simulink model "Project_microgrid_2016"  (R2016a)
settings: Solver=VariableStepAuto  SolverMode=SingleTasking  StartTime=0.0  StopTime=0.3  RelTol=1e-3
undefined symbols (not defined in the file): D1, D11, Delta, DiscIntNeverNeededParam, find_system, Hydride, Metal, Nickel
libraries: powerlib x77, powerlib_meascontrol x31, sps_avr x7, simulink_extras x4, simulink x3, electricdrivelib x1, spsDieselMotorModel x1, re_lib x1
(part 3 of 5)

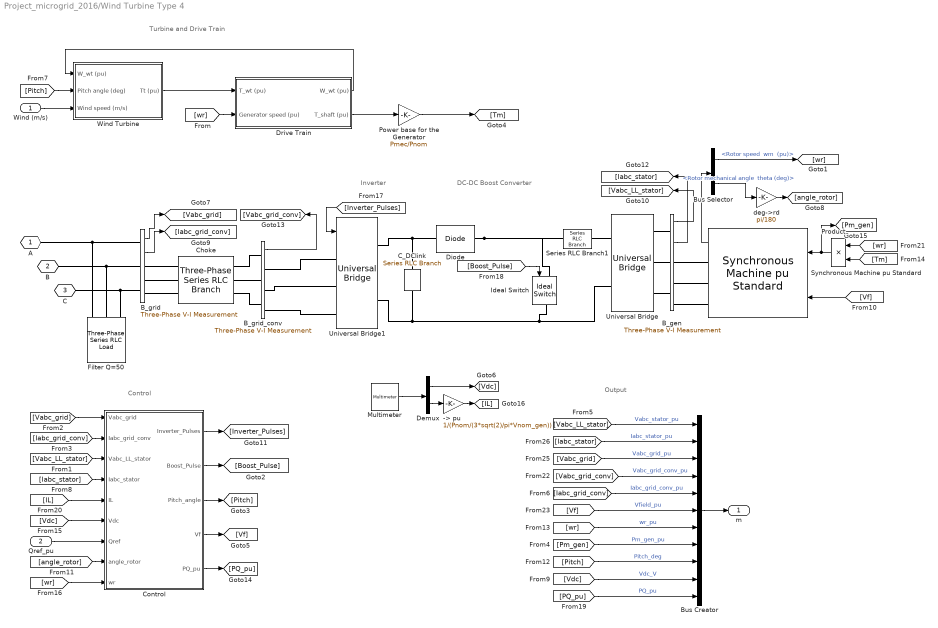
== system Project_microgrid_2016/Wind Turbine Type 4 ==
  note: Turbine and Drive Train
  note: Control
  note: Inverter
  note: DC-DC Boost Converter
  note: Output
  "Wind (m/s) " : Inport
  Qref_pu : Inport  Port=2
  -> pu : Gain  Gain=1/(Pnom/(3*sqrt(2)/pi*Vnom_gen))  SaturateOnIntegerOverflow=on  OutDataTypeStr=Inherit: Same as input  ParamDataTypeStr=Inherit: Same as input
  B_gen : powerlib/Measurements/Three-Phase V-I Measurement  VoltageMeasurement=phase-to-phase  SetLabelV=off  LabelV=Vabc  Vpu=on  VpuLL=off  CurrentMeasurement=yes  SetLabelI=off  LabelI=Iabc  Ipu=on  Pbase=Pnom  Vbase=Vnom_gen  OutputType=Complex  PhasorSimulation=off  PSBequivalent=0
  B_grid : powerlib/Measurements/Three-Phase V-I Measurement  VoltageMeasurement=phase-to-ground  SetLabelV=off  LabelV=Vabc  Vpu=on  VpuLL=off  CurrentMeasurement=yes  SetLabelI=off  LabelI=Iabc  Ipu=on  Pbase=Pnom  Vbase=Vnom  OutputType=Complex  PhasorSimulation=off  PSBequivalent=0
  B_grid_conv : powerlib/Measurements/Three-Phase V-I Measurement  VoltageMeasurement=phase-to-ground  SetLabelV=off  LabelV=Vabc  Vpu=on  VpuLL=off  CurrentMeasurement=no  SetLabelI=off  LabelI=Iabc  Ipu=on  Pbase=Pnom  Vbase=Vnom  OutputType=Complex  PhasorSimulation=off  PSBequivalent=0
  Bus Creator : BusCreator  Inputs=11
  Bus Selector : BusSelector  OutputSignals="Mechanical.Rotor speed  wm  (pu),Mechanical.Rotor mechanical angle  theta (deg)"
  C_DClink : powerlib/Elements/Series RLC Branch  LConnTagsString=__new0  RConnTagsString=__new0  BranchType=C  Resistance=1  Inductance=1e-3  SetiL0=off  InitialCurrent=0  Capacitance=C_DClink  Setx0=on  InitialVoltage=Vdc_nom  Measurements=Branch voltage
  "Choke " : powerlib/Elements/Three-Phase Series RLC Branch  LConnTagsString=A|B|C  RConnTagsString=A|B|C  BranchType=RL  Resistance=R_RL*Vnom^2/Pnom  Inductance=L_RL*Vnom^2/Pnom/(2*pi*Fnom)  Capacitance=[]  Measurements=None
  Control : Subsystem
  Demux : Demux  Outputs=2
  Diode : powerlib/Power Electronics/Diode  Ron=1e-6/Nb_wt  Lon=0  Vf=0  IC=0  UseSnubber=off  Rs=inf  Cs=inf  Measurements=off
  Drive Train : Subsystem  mask(Wind Turbine shaft){H_WT=H_WT, Ksh=Ksh, D_mutual=D_mutual, wbase=2*pi*Fnom/p, w_wt0=w_wt0, torque0=torque0, Ts=Ts}
      mask prompts: H_WT "Wind turbine inertia constant H (s):"; Ksh "Shaft spring constant (pu of nominal mechanical torque/rad):"; D_mutual "Shaft mutual damping (pu of nominal mechanical torque/pu dw):"; wbase "Shaft base speed (rad/s):"; w_wt0 "Turbine initial speed (pu of base speed):"; torque0 "Initial output torque (pu of nominal mechanical torque):"; Ts "Sample time (s):"
      mask help:
      | This block implements a wind turbine drive train model. All shaft parameters are referred to high-speed shaft (generator shaft).
      |
      | The first input is the wind turbine torque in per unit (pu) based on the nominal power of the turbine and the base speed of the generator. The second input is the generator speed in pu based on the base speed of the generator.
      |
      | The outputs are:
      | 1- the transmitted torque of the shaft in pu based on the nominal power of the turbine and the base speed of the generator.
      | 2- the wind turbine speed in pu of the base speed of the generator.
  Filter Q=50 : powerlib/Elements/Three-Phase Series RLC Load  LConnTagsString=A|B|C  Configuration=Y (grounded)  NominalVoltage=Vnom  Vabc=[1e3 1e3 1e3]  Vabcp=[1e3 1e3 1e3]  NominalFrequency=Fnom  UnbalancedPower=off  ActivePower=C_var_filter/Q_filter  InductivePower=0  CapacitivePower=C_var_filter  Pabc=[10e3 9e3 11e3]  QLabc=[100 90 110]  QCabc=[100 90 110]  Pabcp=[10e3 9e3 11e3]  QLabcp=[100 90 110]  QCabcp=[100 90 110]  Measurements=None  LoadType=constant Z
  Ideal Switch : powerlib/Power Electronics/Ideal Switch  Ron=1e-6/Nb_wt  Lon=0  IC=0  Rs=1e5/Nb_wt  Cs=inf  Measurements=off
  Multimeter : powerlib/Measurements/Multimeter  PhasorSimulation=off  OutputType=Complex  sel=[2 3]  L=3  Gain=[1 1]  yselected={'Ub: Wind Turbine Type 4/C_DClink','Ib: Wind Turbine Type 4/Series RLC Branch1'};  PSBOutputType=1  PSBequivalent=0  AxesSetting=[0,0.1,-100,100]  Display=0  SavedBlockNames=-11
  Power base for the Generator : Gain  Gain=Pmec/Pnom  SaturateOnIntegerOverflow=on  OutDataTypeStr=Inherit: Same as input  ParamDataTypeStr=Inherit: Same as input
  Product : Product  RndMeth=Zero
  Series RLC Branch1 : powerlib/Elements/Series RLC Branch  LConnTagsString=__new0  RConnTagsString=__new0  BranchType=RL  Resistance=R_Boost  Inductance=L_Boost  SetiL0=off  InitialCurrent=0  Capacitance=1.0  Setx0=off  InitialVoltage=0  Measurements=Branch current
  Synchronous Machine pu Standard : powerlib/Machines/Synchronous Machine pu Standard  PresetModel=No  MechanicalLoad=Mechanical power Pm  ShowDetailedParameters=on  RotorType=Salient-pole  Units=per unit standard parameters  MeasurementBus=off  NominalParameters="[ Pnom  Vnom_gen Fnom ]"  Reactances1=[ 1.81, 0.3, 0.23, 1.76, 0.65, 0.25, 0.15 ]  Reactances2="[ Xd, Xd1, Xd2, Xq,  Xq2,  Xl ]"  dAxisTimeConstants=Open-circuit  qAxisTimeConstants=Short-circuit  TimeConstants1="[ 4.4849  0.0681  0.1  ]"  TimeConstants2=[ 8.0, 0.03, 1.0, 0.07 ]  TimeConstants3="[  Tdo1  Tdo2  Tq2  ]"  TimeConstants4=[ 8.0, 0.03, 0.3371, 0.0295 ]  TimeConstants5=[ 1.01, 0.053, 0.1 ]  TimeConstants6=[ 1.3201, 0.023, 1.0, 0.07 ]  TimeConstants7="[  1.01  0.053  0.051266  ]"  TimeConstants8=[ 1.3201, 0.0231, 0.3371, 0.0295 ]  StatorResistance=Resistance  Mechanical=[ H F p]  PolePairs=1  InitialConditions=init  SetSaturation=off  Saturation=[0.6404,0.7127,0.8441,0.9214,0.9956,1.082,1.19,1.316,1.457;0.7,0.7698,0.8872,0.9466,0.9969,1.046,1.1,1.151,1.201]  LoadFlowParameters=[1,0,0,0,0]  TsPowergui=0  TsBlock=-1  IterativeModel=Trapezoidal non iterative  IterativeDiscreteModel=Trapezoidal non iterative  BusType=PV  Pref=0  Qref=0  Qmin=-inf  Qmax=inf  PLF=0  QLF=0
  Universal Bridge : powerlib/Power Electronics/Universal Bridge  Arms=3  SnubberResistance=2*Ts_snub/(Pnom/(1000*2*pi*Fnom*Vnom_gen^2))  SnubberCapacitance=Pnom/(1000*2*pi*Fnom*Vnom_gen^2)  Device=Diodes  Ron=1e-6/Nb_wt  Lon=0  ForwardVoltages="[  0  0  ]"  ForwardVoltage=0  GTOparameters=[ 10e-6 , 20e-6 ]  IGBTparameters=[ 1e-6 , 2e-6 ]  Measurements=None  Measurements_2=None  converterType=Rectifier
  Universal Bridge1 : powerlib/Power Electronics/Universal Bridge  Arms=3  SnubberResistance=1e6/Nb_wt  SnubberCapacitance=inf  Device=IGBT / Diodes  Ron=1e-6/Nb_wt  Lon=0  ForwardVoltages="[  0  0  ]"  ForwardVoltage=0  GTOparameters=[ 10e-6 , 20e-6 ]  IGBTparameters=[ 1e-6 , 2e-6 ]*0  Measurements=None  Measurements_2=None  converterType=Rectifier
  Wind Turbine : Subsystem  mask(Wind Turbine){Prated=Pmec, c1_c8=c1_c8, K1_K2=K1_K2, wind0=wind0, Ts=Ts}
      mask prompts: Prated "Nominal mechanical output power (W):"; c1_c8 "Coefficients [c1 ... c8]"; K1_K2 "Parameters [K1 K2]"; wind0 "Initial wind speed (m/s):"; Ts "Sample time (s):"
      mask help:
      | This block implements a generic wind turbine models.
      |
      | The first input is the turbine speed in per unit of the generator base speed. For a synchronous or asynchronous generator, the base speed is the synchronous speed. For a permanent-magnet generator, the base speed is defined as the speed producing nominal voltage at  no load. The second input is the blade pitch angle in degrees. The third input is the wind speed in m/s.
      |
      | The output is the torque applied to the drive train in per unit based on the nominal power of the turbine and the base speed of the generator.
      mask init:
      | c1 = c1_c8(1);
      | c2 = c1_c8(2);
      | c3 = c1_c8(3);
      | c4 = c1_c8(4);
      | c5 = c1_c8(5);
      | c6 = c1_c8(6);
      | c7 = c1_c8(7);;
      | c8 = c1_c8(8);
      | 
      | K1=K1_K2(1);
      | K2=K1_K2(2);
      settings: OpenFcn=power_openblockproxy();
      mask Display: disp('');
  deg->rd : Gain  Gain=pi/180  SaturateOnIntegerOverflow=on  OutDataTypeStr=Inherit: Same as input  ParamDataTypeStr=Inherit: Same as input
  A : PMIOPort  Tag=PMCPort  Side=Left
  B : PMIOPort  Tag=PMCPort  Port=2  Side=Left
  C : PMIOPort  Tag=PMCPort  Port=3  Side=Left
  m : Outport
  wires:
  [Vf] -> Synchronous Machine pu Standard/2
  Wind Turbine/1(Tt (pu)) -> Drive Train/1(T_wt (pu))
  [wr] -> Drive Train/2(Generator speed (pu))
  Drive Train/2(T_shaft (pu)) -> Power base for the Generator/1
  Power base for the Generator/1 -> [Tm]
  "Wind (m/s) "/1 -> Wind Turbine/3(Wind speed (m/s))
  Drive Train/1(W_wt (pu)) -> Wind Turbine/1(W_wt (pu))
  [Pitch] -> Wind Turbine/2(Pitch angle (deg))
  Bus Selector/2 -> deg->rd/1  "<Rotor mechanical angle  theta (deg)>"
  deg->rd/1 -> [angle_rotor]
  Bus Selector/1 -> [wr]  "<Rotor speed  wm  (pu)>"
  [wr] -> Product/1
  Synchronous Machine pu Standard/1 -> Bus Selector/1
  B_grid_conv/1 -> [Vabc_grid_conv]
  [Tm] -> Product/2
  Product/1 -> Synchronous Machine pu Standard/1, [Pm_gen]
  B_grid/1 -> [Vabc_grid]
  B_grid/2 -> [Iabc_grid_conv]
  B_gen/1 -> [Vabc_LL_stator]
  B_gen/2 -> [Iabc_stator]
  [Vabc_grid] -> Control/1(Vabc_grid)
  [Iabc_grid_conv] -> Control/2(Iabc_grid_conv)
  [Vabc_LL_stator] -> Control/3(Vabc_LL_stator)
  [Iabc_stator] -> Control/4(Iabc_stator)
  [Vdc] -> Control/6(Vdc)
  Qref_pu/1 -> Control/7(Qref)
  [angle_rotor] -> Control/8(angle_rotor)
  [wr] -> Control/9(wr)
  Control/1(Inverter_Pulses) -> [Inverter_Pulses]
  Control/2(Boost_Pulse) -> [Boost_Pulse]
  Control/3(Pitch_angle) -> [Pitch]
  Control/4(Vf) -> [Vf]
  [Inverter_Pulses] -> Universal Bridge1/1
  [Boost_Pulse] -> Ideal Switch/1
  Control/5(PQ_pu) -> [PQ_pu]
  [Vabc_LL_stator] -> Bus Creator/1  "Vabc_stator_pu"
  [Iabc_stator] -> Bus Creator/2  "Iabc_stator_pu"
  [Vabc_grid] -> Bus Creator/3  "Vabc_grid_pu"
  Bus Creator/1 -> m/1
  [Vabc_grid_conv] -> Bus Creator/4  "Vabc_grid_conv_pu"
  [Iabc_grid_conv] -> Bus Creator/5  "Iabc_grid_conv_pu"
  [Vf] -> Bus Creator/6  "Vfield_pu"
  [wr] -> Bus Creator/7  "wr_pu"
  [Pm_gen] -> Bus Creator/8  "Pm_gen_pu"
  [Pitch] -> Bus Creator/9  "Pitch_deg"
  [Vdc] -> Bus Creator/10  "Vdc_V"
  [PQ_pu] -> Bus Creator/11  "PQ_pu"
  [IL] -> Control/5(IL)
  Multimeter/1 -> Demux/1
  Demux/1 -> [Vdc]
  Demux/2 -> -> pu/1
  -> pu/1 -> [IL]
  connections:
  B_grid/RConn1 -- "Choke "/LConn1
  B_grid/RConn2 -- "Choke "/LConn2
  B_grid/RConn3 -- "Choke "/LConn3
  A/RConn1 -- B_grid/LConn1 -- Filter Q=50/LConn1
  Filter Q=50/LConn2 -- B_grid/LConn2 -- B/RConn1
  Filter Q=50/LConn3 -- B_grid/LConn3 -- C/RConn1
  "Choke "/RConn1 -- B_grid_conv/LConn1
  "Choke "/RConn2 -- B_grid_conv/LConn2
  "Choke "/RConn3 -- B_grid_conv/LConn3
  Series RLC Branch1/LConn1 -- Universal Bridge/RConn1
  Universal Bridge/LConn1 -- B_gen/LConn1
  Universal Bridge/LConn2 -- B_gen/LConn2
  Universal Bridge/LConn3 -- B_gen/LConn3
  Diode/LConn1 -- Series RLC Branch1/RConn1 -- Ideal Switch/LConn1
  Universal Bridge1/RConn1 -- Diode/RConn1 -- C_DClink/LConn1
  Universal Bridge/RConn2 -- Universal Bridge1/RConn2 -- C_DClink/RConn1 -- Ideal Switch/RConn1
  Synchronous Machine pu Standard/RConn3 -- B_gen/RConn3
  Synchronous Machine pu Standard/RConn2 -- B_gen/RConn2
  Synchronous Machine pu Standard/RConn1 -- B_gen/RConn1
  B_grid_conv/RConn2 -- Universal Bridge1/LConn2
  B_grid_conv/RConn1 -- Universal Bridge1/LConn1
  B_grid_conv/RConn3 -- Universal Bridge1/LConn3

== system Project_microgrid_2016/Battery/Subsystem4 ==
  "  " : powerlib/Measurements/Voltage Measurement  PhasorSimulation=off  OutputType=Complex  PSBequivalent=0
  "    " : powerlib/Elements/Series RLC Branch  LConnTagsString=__new0  RConnTagsString=__new0  BranchType=RC  Resistance=0  Inductance=69e-3  SetiL0=off  InitialCurrent=0  Capacitance=9.6e-7  Setx0=off  InitialVoltage=0  Measurements=None
  " Measurement" : powerlib/Measurements/Voltage Measurement  PhasorSimulation=off  OutputType=Complex  PSBequivalent=0
  " Measurement1" : powerlib/Measurements/Current Measurement  PhasorSimulation=off  OutputType=Complex  PSBequivalent=0
  Diode : powerlib/Power Electronics/Diode  Ron=0.001  Lon=0  Vf=0.8  IC=0  UseSnubber=off  Rs=500  Cs=250e-9  Measurements=on
  Mosfet : powerlib/Power Electronics/Mosfet  Ron=0.1  Lon=0  Rd=0.01  Vfd=0  IC=0  Rs=1e5  Cs=inf  Measurements=on
  Pulse Generator : DiscretePulseGenerator  PulseType=Time based  Period=1/100000  PulseWidth=50
  Scope : Scope  NumInputPorts=2
  Series RLC Branch : powerlib/Elements/Series RLC Branch  LConnTagsString=__new0  RConnTagsString=__new0  BranchType=RL  Resistance=0  Inductance=2.332e-3  SetiL0=off  InitialCurrent=0  Capacitance=1e-6  Setx0=off  InitialVoltage=0  Measurements=None
  + : PMIOPort  Side=Left
  _ : PMIOPort  Port=2  Side=Left
  ++ : PMIOPort  Port=3  Side=Right
  __ : PMIOPort  Port=4  Side=Right
  wires:
  Pulse Generator/1 -> Mosfet/1
  "  "/1 -> Scope/1
  " Measurement"/1 -> Scope/2
  connections:
  "  "/LConn1 -- Series RLC Branch/LConn1 -- +/RConn1
  Diode/RConn1 -- " Measurement1"/LConn1 -- "    "/LConn1
  ++/RConn1 -- " Measurement"/LConn1 -- " Measurement1"/RConn1
  Mosfet/RConn1 -- _/RConn1 -- "  "/LConn2 -- "    "/RConn1 -- __/RConn1 -- " Measurement"/LConn2
  Series RLC Branch/RConn1 -- Mosfet/LConn1 -- Diode/LConn1

== system Project_microgrid_2016/Diesle Generator/EXCITATION ==
  Vref : Inport
  Vt : Inport  Port=2
  It : Inport  Port=3
  Ifd : Inport  Port=4
  Vstab : Inport  Port=5
  AC1A : Subsystem  VariantControl=Variant1
  AC4A : Subsystem  VariantControl=Variant2
  AC5A : Subsystem  VariantControl=Variant3
  DC1A : Subsystem  VariantControl=Variant4
  DC2A : Subsystem  VariantControl=Variant5
  ST1A : Subsystem  VariantControl=Variant6
  ST2A : sps_avr/ST2A Excitation System  VariantControl=Variant7  Tr=20e-3  KaTa=[120 0.15]  VRminmax=[0 1.0]  KfTf=[0.05 1.0]  KeTe=[1.0 0.5]  KI=8.0  Kp=4.88  Xd=1.56  Kc=1.82  v0=[1,1.42734]  I0=0.2739  TsBlock=-2
  Efd : Outport

== system Project_microgrid_2016/Inveter/VSC Contoler ==
  VSC Control : Subsystem  mask(VSC Main Controller){nom=[ 7500  50 ], Vnom=[ 25e3 260 ], Vnom_dc=600, RLxfo=[0.002  0.06 ], RLchoke=[2e-3  250e-6  ], K_VDCreg=[7  800], K_Ireg=[0.3 20], Ts=0.0001}
      mask prompts: nom "Nominal power and frequency [ Pnom(VA)  Fnom(Hz) ]:"; Vnom "Nominal primary and secondary voltages (Vrms LL) [ Vnom_prim   Vnom_sec ]:"; Vnom_dc "Nominal DC bus voltage (V):"; RLxfo "Total transformer leakage impedance (pu/Pnom) [ Rxfo  Lxf ]"; RLchoke "Choke impedance [ R(ohm) L(H) ]"; K_VDCreg "VDC regultator gains [ Kp  Ki ]:"; K_Ireg "Current regulator gains [ Kp  Ki ]:"; Ts "Sample time"
      mask init:
      | Pnom=nom(1);
      | Fnom=nom(2);
      | Vnom_prim=Vnom(1);
      | Vnom_sec=Vnom(2);
      | Zbase=Vnom_sec^2/Pnom;
      | Rtot_pu=RLxfo(1) + RLchoke(1)/Zbase;
      | Ltot_pu=RLxfo(2) + RLchoke(2)/(Zbase/(2*pi*Fnom));
      | Kp_VDCreg=K_VDCreg(1);
      | Ki_VDCreg=K_VDCreg(2);
      | Kp_Ireg=K_Ireg(1);
      | Ki_Ireg=K_Ireg(2);
      | Vdc_ref=Vnom_dc;
      | % Used to determine initial value of Boost Control (MPPT)
      | assignin('base','Vdc_ref_Inv',Vdc_ref);
  Inveter Pulse : Outport
  wires:
  [Vabc_B1] -> VSC Control/1(Vabc_prim)
  [Iabc_B1] -> VSC Control/2(Iabc_prim)
  [Vdc] -> VSC Control/3(Vdc_mes)
  VSC Control/1(Pulses) -> Inveter Pulse/1

== system Project_microgrid_2016/Relay G/AC Time Overcurrent Relay2 ==
  I : Inport
  Clock : Clock
  Irms : powerlib_meascontrol/Measurements/RMS  TrueRMS=on  Freq=Freq  RMSInit=RMSInit  Ts=0
  Relational Operator : RelationalOperator  Operator=<=  OutDataTypeStr=boolean
  Time Relay Function : MATLAB Function  TreatAsAtomicUnit=on
  C.B : Outport
  OT : Outport  Port=2
  wires:
  Clock/1 -> Relational Operator/1, Time Relay Function/1(clk)
  Irms/1 -> Time Relay Function/2(Irms)
  Time Relay Function/1(TT) -> Relational Operator/2
  Time Relay Function/2(OT) -> OT/1
  Relational Operator/1 -> C.B/1
  I/1 -> Irms/1

== system Project_microgrid_2016/Relay G/Output1 ==
  Signal : Inport
  Demux : Demux  Outputs=3
  Scope : Scope  NumInputPorts=3
  wires:
  Demux/3 -> Scope/3
  Demux/1 -> Scope/1
  Demux/2 -> Scope/2
  Signal/1 -> Demux/1

== system Project_microgrid_2016/Relay PV/AC Time Overcurrent Relay2 ==
  I : Inport
  Clock : Clock
  Irms : powerlib_meascontrol/Measurements/RMS  TrueRMS=on  Freq=Freq  RMSInit=RMSInit  Ts=0
  Relational Operator : RelationalOperator  Operator=<=  OutDataTypeStr=boolean
  Time Relay Function : MATLAB Function  TreatAsAtomicUnit=on
  C.B : Outport
  OT : Outport  Port=2
  wires:
  Clock/1 -> Relational Operator/1, Time Relay Function/1(clk)
  Irms/1 -> Time Relay Function/2(Irms)
  Time Relay Function/1(TT) -> Relational Operator/2
  Time Relay Function/2(OT) -> OT/1
  Relational Operator/1 -> C.B/1
  I/1 -> Irms/1

== system Project_microgrid_2016/Relay W/AC Time Overcurrent Relay2 ==
  I : Inport
  Clock : Clock
  Irms : powerlib_meascontrol/Measurements/RMS  TrueRMS=on  Freq=Freq  RMSInit=RMSInit  Ts=0
  Relational Operator : RelationalOperator  Operator=<=  OutDataTypeStr=boolean
  Time Relay Function : MATLAB Function  TreatAsAtomicUnit=on
  C.B : Outport
  OT : Outport  Port=2
  wires:
  Clock/1 -> Relational Operator/1, Time Relay Function/1(clk)
  Irms/1 -> Time Relay Function/2(Irms)
  Time Relay Function/1(TT) -> Relational Operator/2
  Time Relay Function/2(OT) -> OT/1
  Relational Operator/1 -> C.B/1
  I/1 -> Irms/1

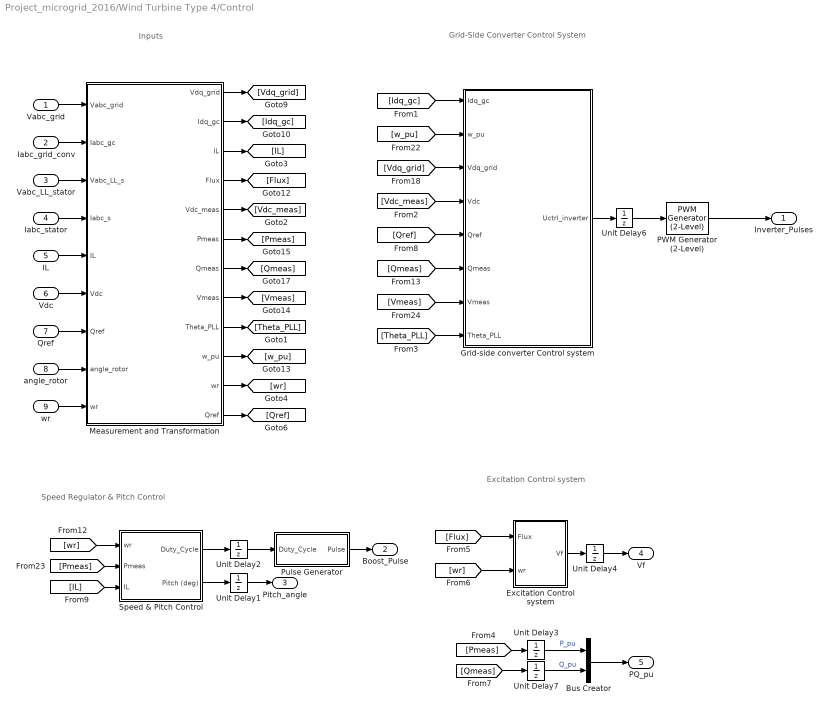
== system Project_microgrid_2016/Wind Turbine Type 4/Control ==
  note: Inputs
  note: Grid-Side Converter
      | Control System
  note: Speed Regulator & Pitch Control
  note: Excitation
      | Control system
  Vabc_grid : Inport
  Iabc_grid_conv : Inport  Port=2
  Vabc_LL_stator : Inport  Port=3
  Iabc_stator : Inport  Port=4
  IL : Inport  Port=5
  Vdc : Inport  Port=6
  Qref : Inport  Port=7
  angle_rotor : Inport  Port=8
  wr : Inport  Port=9
  Bus Creator : BusCreator  Inputs=2
  Excitation Control system : Subsystem
  Grid-side converter Control system : Subsystem
  Measurement and Transformation : Subsystem
  PWM Generator (2-Level) : powerlib_meascontrol/Pulse & Signal Generators/PWM Generator (2-Level)  ModulatorType=Three-phase bridge (6 pulses)  ModulatorMode=Unsynchronized  Fc=Freq_PWM  Pc=90  nF=27  MinMax="[ -1  1 ]"  SamplingTechnique=Natural  ModulatingSignals=off  m=0.8  Freq=60  Phase=0  Ts=Ts  ShowCarrierOutport=off
  Pulse Generator : Subsystem  mask{Freq_sawtooth=Freq_sawtooth, Ts=Ts}
      mask prompts: Freq_sawtooth "Frequency of the carrier (sawtooth signal) (Hz):"; Ts "Sample time (Ts) (s):"
  Speed & Pitch Control : Subsystem
  Unit Delay{1..4,6..7} (6 alike) : UnitDelay  SampleTime=Ts  HasFrameUpgradeWarning=on
  Inverter_Pulses : Outport
  Boost_Pulse : Outport  Port=2
  Pitch_angle : Outport  Port=3
  Vf : Outport  Port=4
  PQ_pu : Outport  Port=5
  wires:
  Excitation Control system/1(Vf) -> Unit Delay4/1
  Speed & Pitch Control/2(Pitch (deg)) -> Unit Delay1/1
  [Idq_gc] -> Grid-side converter Control system/1(Idq_gc)
  [w_pu] -> Grid-side converter Control system/2(w_pu)
  [Vdq_grid] -> Grid-side converter Control system/3(Vdq_grid)
  [Vdc_meas] -> Grid-side converter Control system/4(Vdc)
  [Qref] -> Grid-side converter Control system/5(Qref)
  [Qmeas] -> Grid-side converter Control system/6(Qmeas)
  [Vmeas] -> Grid-side converter Control system/7(Vmeas)
  Speed & Pitch Control/1(Duty_Cycle) -> Unit Delay2/1
  [Flux] -> Excitation Control system/1(Flux)
  [wr] -> Excitation Control system/2(wr)
  [Theta_PLL] -> Grid-side converter Control system/8(Theta_PLL)
  Unit Delay2/1 -> Pulse Generator/1(Duty_Cycle)
  Unit Delay1/1 -> Pitch_angle/1
  Unit Delay4/1 -> Vf/1
  PWM Generator (2-Level)/1 -> Inverter_Pulses/1
  Grid-side converter Control system/1(Uctrl_inverter) -> Unit Delay6/1
  Pulse Generator/1(Pulse) -> Boost_Pulse/1
  Unit Delay6/1 -> PWM Generator (2-Level)/1
  Bus Creator/1 -> PQ_pu/1
  [Pmeas] -> Unit Delay3/1
  [Qmeas] -> Unit Delay7/1
  Unit Delay3/1 -> Bus Creator/1  "P_pu"
  Unit Delay7/1 -> Bus Creator/2  "Q_pu"
  [wr] -> Speed & Pitch Control/1(wr)
  [Pmeas] -> Speed & Pitch Control/2(Pmeas)
  [IL] -> Speed & Pitch Control/3(IL)
  Vabc_grid/1 -> Measurement and Transformation/1(Vabc_grid)
  Iabc_grid_conv/1 -> Measurement and Transformation/2(Iabc_gc)
  Vabc_LL_stator/1 -> Measurement and Transformation/3(Vabc_LL_s)
  Iabc_stator/1 -> Measurement and Transformation/4(Iabc_s)
  IL/1 -> Measurement and Transformation/5(IL)
  Vdc/1 -> Measurement and Transformation/6(Vdc)
  Qref/1 -> Measurement and Transformation/7(Qref)
  angle_rotor/1 -> Measurement and Transformation/8(angle_rotor)
  wr/1 -> Measurement and Transformation/9(wr)
  Measurement and Transformation/1(Vdq_grid) -> [Vdq_grid]
  Measurement and Transformation/2(Idq_gc) -> [Idq_gc]
  Measurement and Transformation/3("IL ") -> [IL]
  Measurement and Transformation/4(Flux) -> [Flux]
  Measurement and Transformation/5(Vdc_meas) -> [Vdc_meas]
  Measurement and Transformation/6(Pmeas) -> [Pmeas]
  Measurement and Transformation/7(Qmeas) -> [Qmeas]
  Measurement and Transformation/8(Vmeas) -> [Vmeas]
  Measurement and Transformation/9(Theta_PLL) -> [Theta_PLL]
  Measurement and Transformation/10(w_pu) -> [w_pu]
  Measurement and Transformation/11("wr ") -> [wr]
  Measurement and Transformation/12("Qref ") -> [Qref]

== system Project_microgrid_2016/Wind Turbine Type 4/Drive Train ==
  note: Wind turbine drive train based on a 2-masse model
  note: Turbine
  note: Shaft
  T_wt (pu) : Inport
  Generator speed (pu) : Inport  Port=2
  1_2H_WT : Gain  Gain=1/(2*H_WT)  SaturateOnIntegerOverflow=on  OutDataTypeStr=Inherit: Same as input  ParamDataTypeStr=Inherit: Same as input
  Discrete-Time Integrator : DiscreteIntegrator  InitialCondition=w_wt0  SampleTime=Ts  ICPrevOutput=DiscIntNeverNeededParam  ICPrevScaledInput=DiscIntNeverNeededParam
  Discrete-Time Integrator1 : DiscreteIntegrator  InitialCondition=torque0/Ksh  SampleTime=Ts  ICPrevOutput=DiscIntNeverNeededParam  ICPrevScaledInput=DiscIntNeverNeededParam
  Mutual damping : Gain  Gain=D_mutual  SaturateOnIntegerOverflow=on  OutDataTypeStr=Inherit: Same as input  ParamDataTypeStr=Inherit: Same as input
  Stiffness : Gain  Gain=Ksh  SaturateOnIntegerOverflow=on  OutDataTypeStr=Inherit: Same as input  ParamDataTypeStr=Inherit: Same as input
  Sum : Sum  Inputs=+-  SaturateOnIntegerOverflow=on  InputSameDT=on  OutDataTypeStr=Inherit: Same as first input
  Sum1 : Sum  Inputs=+-  SaturateOnIntegerOverflow=on  InputSameDT=on  OutDataTypeStr=Inherit: Same as first input
  Sum2 : Sum  SaturateOnIntegerOverflow=on  InputSameDT=on  OutDataTypeStr=Inherit: Same as first input
  wbase : Gain  Gain=wbase  SaturateOnIntegerOverflow=on  OutDataTypeStr=Inherit: Same as input  ParamDataTypeStr=Inherit: Same as input
  W_wt (pu) : Outport
  T_shaft (pu) : Outport  Port=2
  wires:
  T_wt (pu)/1 -> Sum/1
  Sum2/1 -> T_shaft (pu)/1, Sum/2
  Mutual damping/1 -> Sum2/2
  Sum1/1 -> Mutual damping/1, wbase/1
  Generator speed (pu)/1 -> Sum1/2
  Discrete-Time Integrator/1 -> W_wt (pu)/1, Sum1/1
  1_2H_WT/1 -> Discrete-Time Integrator/1
  Sum/1 -> 1_2H_WT/1
  Stiffness/1 -> Sum2/1
  Discrete-Time Integrator1/1 -> Stiffness/1
  wbase/1 -> Discrete-Time Integrator1/1

== system Project_microgrid_2016/Wind Turbine Type 4/Wind Turbine ==
  W_wt (pu) : Inport
  Pitch angle (deg) : Inport  Port=2
  Wind speed (m/s) : Inport  Port=3
  ->pu : Gain  Gain=1/Prated
  Avoid div. by zero : Saturate  UpperLimit=inf  LowerLimit=eps
  "Avoid div. by zero " : Saturate  UpperLimit=inf  LowerLimit=eps
  Fcn1 : Fcn  Expr=K1*u[2]/u[1]
  Fcn2 : Fcn  Expr=c1*(c6*u[1] + (-c4 - c3*(2.5 + u[2]) + c2*(1/(u[1] + c7*(2.5 + u[2])) -c8/(1 + (2.5 + u[2])^3)))/exp(c5*(1/(u[1] + c7*(2.5 + u[2])) - c8/(1 + (2.5 + u[2])^3))))
  "K2*Cp*wind^3 " : Fcn  Expr=K2*u[1]^3*u[2]
  Mux : Mux  Inputs=2
  Mux1 : Mux  Inputs=2
  Mux2 : Mux  Inputs=2
  Product2 : Product  Inputs=*/  SaturateOnIntegerOverflow=on  InputSameDT=on  OutDataTypeStr=Inherit: Same as first input
  Tt (pu) : Outport
  wires:
  ->pu/1 -> Product2/1  "power_pu"
  Product2/1 -> Tt (pu)/1
  Wind speed (m/s)/1 -> Avoid div. by zero/1
  Fcn1/1 -> Mux1/1  "lambda"
  Mux1/1 -> Fcn2/1
  Mux/1 -> Fcn1/1
  Fcn2/1 -> Mux2/2  "Cp"
  Mux2/1 -> "K2*Cp*wind^3 "/1
  Pitch angle (deg)/1 -> Mux1/2
  W_wt (pu)/1 -> "Avoid div. by zero "/1
  Avoid div. by zero/1 -> Mux2/1, Mux/1
  "Avoid div. by zero "/1 -> Mux/2, Product2/2
  "K2*Cp*wind^3 "/1 -> ->pu/1

== system Project_microgrid_2016/Diesle Generator/EXCITATION/AC1A ==
  Vref : Inport
  Vt : Inport  Port=2
  It : Inport  Port=3
  Ifd : Inport  Port=4
  Vstab : Inport  Port=5
  AC1A : sps_avr/AC1A Excitation System  Tr=20e-3  KaTa=[400 0.02]  VAminmax=[-14.5 14.5]  VRminmax=[-5.43 6.03]  KfTf=[0.03 1.0]  TbTc=[0 0]  KeTe=[1.0 0.80]  Ve12=[4.18 3.14]  SeVe12=[0.10 0.03]  Kd=0.38  Kc=0.20  v0=[1 1.4273]  TsBlock=-2
  term3 : Terminator
  Efd : Outport
  wires:
  It/1 -> term3/1
  AC1A/1 -> Efd/1
  Vstab/1 -> AC1A/4
  Ifd/1 -> AC1A/3
  Vt/1 -> AC1A/2
  Vref/1 -> AC1A/1

== system Project_microgrid_2016/Diesle Generator/EXCITATION/AC4A ==
  Vref : Inport
  Vt : Inport  Port=2
  It : Inport  Port=3
  Ifd : Inport  Port=4
  Vstab : Inport  Port=5
  AC4A : sps_avr/AC4A Excitation System  Tr=20e-3  KaTa=[200 0.015]  VIminmax=[-10 10]  VRminmax=[-4.53 5.64]  TbTc=[10 1.0]  Kc=0  v0=[1,1.42734]  TsBlock=-2
  term3 : Terminator
  Efd : Outport
  wires:
  It/1 -> term3/1
  AC4A/1 -> Efd/1
  Vstab/1 -> AC4A/4
  Ifd/1 -> AC4A/3
  Vt/1 -> AC4A/2
  Vref/1 -> AC4A/1

== system Project_microgrid_2016/Diesle Generator/EXCITATION/AC5A ==
  Vref : Inport
  Vt : Inport  Port=2
  It : Inport  Port=3
  Ifd : Inport  Port=4
  Vstab : Inport  Port=5
  AC5A : sps_avr/AC5A Excitation System  Tr=20e-3  KaTa=[100 0.02]  VRminmax=[-7.3 7.3]  KfTf=[0.03 1 0 0]  KeTe=[1.0 0.02]  Efd12=[5.6 0.75*5.6]  SeEfd12=[0.86 0.5]  v0=[1,1.42734]  TsBlock=-2
  term3 : Terminator
  term4 : Terminator
  Efd : Outport
  wires:
  Ifd/1 -> term4/1
  It/1 -> term3/1
  AC5A/1 -> Efd/1
  Vstab/1 -> AC5A/3
  Vt/1 -> AC5A/2
  Vref/1 -> AC5A/1

== system Project_microgrid_2016/Diesle Generator/EXCITATION/DC1A ==
  Vref : Inport
  Vt : Inport  Port=2
  It : Inport  Port=3
  Ifd : Inport  Port=4
  Vstab : Inport  Port=5
  DC1A : sps_avr/DC1A Excitation System  Tr=20e-3  KaTa=[46 0.06]  VRminmax=[-0.9 1.0]  KfTf=[0.05 1.5]  TbTc=[0 0]  KeTe=[0.05 0.46]  Efd12=[3.1 2.3]  SeEfd12=[0.33 0.10]  v0=[1,1.42734]  TsBlock=-2
  term3 : Terminator
  term4 : Terminator
  Efd : Outport
  wires:
  Ifd/1 -> term4/1
  It/1 -> term3/1
  DC1A/1 -> Efd/1
  Vstab/1 -> DC1A/3
  Vt/1 -> DC1A/2
  Vref/1 -> DC1A/1

== system Project_microgrid_2016/Diesle Generator/EXCITATION/DC2A ==
  Vref : Inport
  Vt : Inport  Port=2
  It : Inport  Port=3
  Ifd : Inport  Port=4
  Vstab : Inport  Port=5
  DC2A : sps_avr/DC2A Excitation System  Tr=20e-3  KaTa=[46 0.06]  VRminmax=[-4.9 4.95]  KfTf=[0.05 1.5]  TbTc=[0 0]  KeTe=[0.05 0.46]  Efd12=[3.05 2.29]  SeEfd12=[0.279 0.117]  v0=[1,1.42734]  TsBlock=-2
  term3 : Terminator
  term4 : Terminator
  Efd : Outport
  wires:
  Ifd/1 -> term4/1
  It/1 -> term3/1
  DC2A/1 -> Efd/1
  Vstab/1 -> DC2A/3
  Vt/1 -> DC2A/2
  Vref/1 -> DC2A/1

== system Project_microgrid_2016/Diesle Generator/EXCITATION/ST1A ==
  Vref : Inport
  Vt : Inport  Port=2
  It : Inport  Port=3
  Ifd : Inport  Port=4
  Vstab : Inport  Port=5
  ST1A : sps_avr/ST1A Excitation System  Tr=20e-3  KaTa=[210 0.001]  VIminmax=[-999 999]  VAminmax=[-999 999]  VRminmax=[-6.0 6.43]  KfTf=[0.001 1]  TbTc=[0 0 0 0]  KLR=1  ILR=2  Kc=0.038  v0=[1,1.42734]  TsBlock=-2
  term3 : Terminator
  Efd : Outport
  wires:
  It/1 -> term3/1
  ST1A/1 -> Efd/1
  Vstab/1 -> ST1A/4
  Ifd/1 -> ST1A/3
  Vt/1 -> ST1A/2
  Vref/1 -> ST1A/1

== system Project_microgrid_2016/Inveter/VSC Contoler/VSC Control ==
  note: VSC Main Controller
  Vabc_prim : Inport  PortDimensions=3
  Iabc_prim : Inport  Port=2  PortDimensions=3
  Vdc_mes : Inport  Port=3  PortDimensions=1
  Current Regulator : Subsystem
  Deblock Converters1 : Step  Time=0.05  SampleTime=0
  Iq_ref : Constant  Value=0
  Mux : Mux  Inputs=2
  PLL & Measurements : Subsystem
  PWM Generator (3-Level) : powerlib_meascontrol/Pulse & Signal Generators/PWM Generator (3-Level)  ModulatorType=Three-phase bridge (12 pulses)  ModulatorMode=Unsynchronized  nF=27  Fc=33*60  ModulatingSignals=off  m=0.8  Freq=60  Phase=0  Ts=1e-6
  Product1 : Product  RndMeth=Zero
  Uabc_ref Generation max (m) = 1 : Subsystem
  Unit Delay : UnitDelay  SampleTime=0.0001  HasFrameUpgradeWarning=on
  VDC Regulator : Subsystem
  Vdc_ref1 : Constant  Value=Vdc_ref
  Pulses : Outport
  wires:
  VDC Regulator/1(Id_ref) -> Mux/1
  PLL & Measurements/1(wt) -> Uabc_ref Generation max (m) = 1/1(wt)
  Current Regulator/1(VdVq_conv) -> Uabc_ref Generation max (m) = 1/2(VdVq_conv)
  Iq_ref/1 -> Mux/2
  Mux/1 -> Current Regulator/3(IdIq_ref)
  PLL & Measurements/3(IdIq_prim) -> Current Regulator/2(IdIq_mes)
  PLL & Measurements/2(VdVq_prim) -> Current Regulator/1(VdVq_mes)
  Vdc_mes/1 -> VDC Regulator/1(Vdc_mes)
  Vabc_prim/1 -> PLL & Measurements/1(Vabc_prim)
  Iabc_prim/1 -> PLL & Measurements/2(Iabc_prim)
  Unit Delay/1 -> PWM Generator (3-Level)/1
  Uabc_ref Generation max (m) = 1/1(Uabc_ref) -> Unit Delay/1
  Vdc_ref1/1 -> VDC Regulator/2(Vdc_ref)
  Deblock Converters1/1 -> Product1/1
  Product1/1 -> Pulses/1
  PWM Generator (3-Level)/1 -> Product1/2

== system Project_microgrid_2016/Wind Turbine Type 4/Control/Excitation Control system ==
  Flux : Inport
  wr : Inport  Port=2
  Discrete PI Controller : Subsystem  DialogController=POWERSYS.PowerSysDialog  mask(Discrete PI Controller){Kp=Kp_field, Ki=Ki_field, Par_Limits=[1 0]*Vf_limit, Init=init(9), Ts=Ts}
      mask prompts: Kp "Proportional gain (Kp):"; Ki "Integral gain (Ki):"; Par_Limits "Output limits: [ Upper   Lower ]"; Init "Output initial value:"; Ts "Sample time:"
      mask help: This block implements a discrete PI controller.
      mask init:
      | UpperLimit=Par_Limits(1);
      | LowerLimit=Par_Limits(2);
      | power_initmask();
      mask Help: This block is part of a subset of blocks in the Extras library that does not have documentation associated with it, other than the block mask description.
      mask Display: disp('PI');
  Divide : Product  Inputs=*/
  Flux_ref : Constant
  "Flux_ref " : Constant
  Sum4 : Sum  Inputs=|+-  SaturateOnIntegerOverflow=on  InputSameDT=on  OutDataTypeStr=Inherit: Same as first input
  Switch : Switch  Threshold=1
  avoid division by 0 : Saturate  UpperLimit=inf  LowerLimit=1e-6
  Vf : Outport
  wires:
  Switch/1 -> Sum4/1
  Divide/1 -> Switch/1
  avoid division by 0/1 -> Divide/2
  "Flux_ref "/1 -> Divide/1
  Flux_ref/1 -> Switch/3
  wr/1 -> avoid division by 0/1, Switch/2
  Flux/1 -> Sum4/2  "Flux"
  Discrete PI Controller/1(Out) -> Vf/1  "Vf"
  Sum4/1 -> Discrete PI Controller/1(Error)

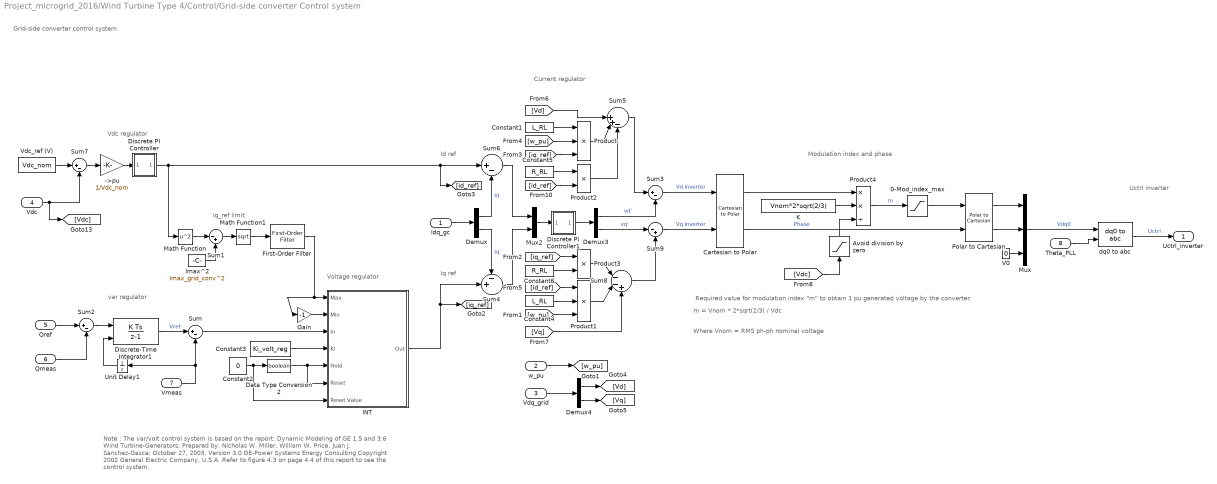
== system Project_microgrid_2016/Wind Turbine Type 4/Control/Grid-side converter Control system ==
  note: Note :
      | The var/volt control system is based on the report:
      | Dynamic Modeling of GE 1.5 and 3.6 Wind Turbine-Generators;
      | Prepared by: Nicholas W. Miller, William W. Price, Juan J. Sanchez-Gasca;
      | October 27, 2003, Version 3.0
      | GE-Power Systems Energy Consulting
      | Copyright 2002 General Electric Company, U.S.A.
      |
      | Refer to figure 4.3 on page 4.4 of this report to see the control system.
  note: Uctrl inverter
  note: Modulation index and phase
  note: Where Vnom = RMS ph-ph nominal voltage
  note: m = Vnom * 2*sqrt(2/3) / Vdc
  note: Required value for modulation index "m" to obtain 1 pu generated voltage by the converter:
  note: Iq ref
  note: Id ref
  note: Current regulator
  note: Iq_ref limit
  note: Vdc regulator
  note: Voltage regulator
  note: var regulator
  note: Grid-side converter control system
  Idq_gc : Inport
  w_pu : Inport  Port=2
  Vdq_grid : Inport  Port=3
  Vdc : Inport  Port=4
  Qref : Inport  Port=5
  Qmeas : Inport  Port=6
  Vmeas : Inport  Port=7
  Theta_PLL : Inport  Port=8
  ->pu : Gain  Gain=1/Vdc_nom
  0-Mod_index_max : Saturate  UpperLimit=Mod_index_max  LowerLimit=0
  Avoid division by zero : Saturate  UpperLimit=1e6  LowerLimit=1e-6
  Cartesian to Polar : simulink_extras/Transformations/Cartesian to Polar
  Constant1 : Constant  Value=L_RL
  Constant2 : Constant  Value=0
  Constant3 : Constant  Value=Ki_volt_reg
  Constant4 : Constant  Value=L_RL
  Constant5 : Constant  Value=R_RL
  Constant6 : Constant  Value=R_RL
  Data Type Conversion2 : DataTypeConversion  OutDataTypeStr=boolean
  Demux : Demux  Outputs=2
  Demux3 : Demux  Outputs=2
  Demux4 : Demux  Outputs=2
  Discrete PI Controller : Subsystem  DialogController=POWERSYS.PowerSysDialog  mask(Discrete PI Controller){Kp=Kp_dc, Ki=Ki_dc, Par_Limits=[1 -1]*Imax_grid_conv, Init=0, Ts=Ts}
      mask prompts: Kp "Proportional gain (Kp):"; Ki "Integral gain (Ki):"; Par_Limits "Output limits: [ Upper   Lower ]"; Init "Output initial value:"; Ts "Sample time:"
      mask help: This block implements a discrete PI controller.
      mask init:
      | UpperLimit=Par_Limits(1);
      | LowerLimit=Par_Limits(2);
      | power_initmask();
      mask Help: This block is part of a subset of blocks in the Extras library that does not have documentation associated with it, other than the block mask description.
      mask Display: disp('PI');
  Discrete PI Controller1 : Subsystem  DialogController=POWERSYS.PowerSysDialog  mask(Discrete PI Controller){Kp=Kp_grid_side_cur_reg, Ki=Ki_grid_side_cur_reg, Par_Limits=[1 -1]*Current_reg_output_limit, Init=0, Ts=Ts}
      mask prompts: Kp "Proportional gain (Kp):"; Ki "Integral gain (Ki):"; Par_Limits "Output limits: [ Upper   Lower ]"; Init "Output initial value:"; Ts "Sample time:"
      mask help: This block implements a discrete PI controller.
      mask init:
      | UpperLimit=Par_Limits(1);
      | LowerLimit=Par_Limits(2);
      | power_initmask();
      mask Help: This block is part of a subset of blocks in the Extras library that does not have documentation associated with it, other than the block mask description.
      mask Display: disp('PI');
  Discrete-Time Integrator1 : DiscreteIntegrator  gainval=Ki_var_reg  InitialConditionSource=external  InitialCondition=1  SampleTime=Ts  LimitOutput=on  UpperSaturationLimit=Var_reg_output_hi_limit  LowerSaturationLimit=Var_reg_output_low_limit  ICPrevOutput=DiscIntNeverNeededParam  ICPrevScaledInput=DiscIntNeverNeededParam
  First-Order Filter : powerlib_meascontrol/Filters/First-Order Filter  FilterType=Lowpass  Tc=Iq_ref_limit_time_constant  Ts=Ts  Initialize=on  Vac_Init=[0, 0, 0]  Vdc_Init=Imax_grid_conv  PlotResponse=off  FreqRange="[0,  200,  1]"
  Gain : Gain  Gain=-1  SaturateOnIntegerOverflow=on  OutDataTypeStr=Inherit: Same as input  ParamDataTypeStr=Inherit: Same as input
  INT : Subsystem  mask(Integrator  With  External  Dynamic  Limits (Discrete)){}
      mask Display: disp('Discrete-Time\n(Trapezoidal)\nIntegrator\n ')
  Imax^2 : Constant  Value=Imax_grid_conv^2
  K : Constant  Value=Vnom*2*sqrt(2/3)
  Math Function : Math  Operator=square  SaturateOnIntegerOverflow=on
  Math Function1 : Math  Operator=sqrt  SaturateOnIntegerOverflow=on
  Mux : Mux  Inputs=3
  Mux2 : Mux  Inputs=2
  Polar to Cartesian : simulink_extras/Transformations/Polar to Cartesian
  Product : Product  Inputs=3  SaturateOnIntegerOverflow=on  InputSameDT=on  OutDataTypeStr=Inherit: Same as first input
  Product1 : Product  Inputs=3  SaturateOnIntegerOverflow=on  InputSameDT=on  OutDataTypeStr=Inherit: Same as first input
  Product2 : Product  SaturateOnIntegerOverflow=on  InputSameDT=on  OutDataTypeStr=Inherit: Same as first input
  Product3 : Product  SaturateOnIntegerOverflow=on  InputSameDT=on  OutDataTypeStr=Inherit: Same as first input
  Product4 : Product  Inputs=**/  SaturateOnIntegerOverflow=on  InputSameDT=on  OutDataTypeStr=Inherit: Same as first input
  Sum{,2..3,6..7} (5 alike) : Sum  Inputs=|+-  SaturateOnIntegerOverflow=on  InputSameDT=on  OutDataTypeStr=Inherit: Same as first input
  Sum1 : Sum  Inputs=|-+  SaturateOnIntegerOverflow=on  InputSameDT=on  OutDataTypeStr=Inherit: Same as first input
  Sum4 : Sum  Inputs=-+|  SaturateOnIntegerOverflow=on  InputSameDT=on  OutDataTypeStr=Inherit: Same as first input
  Sum5 : Sum  Inputs=||++-  SaturateOnIntegerOverflow=on  InputSameDT=on  OutDataTypeStr=Inherit: Same as first input
  Sum8 : Sum  Inputs=|--+  SaturateOnIntegerOverflow=on  InputSameDT=on  OutDataTypeStr=Inherit: Same as first input
  Sum9 : Sum  Inputs=|-+  SaturateOnIntegerOverflow=on  InputSameDT=on  OutDataTypeStr=Inherit: Same as first input
  Unit Delay1 : UnitDelay  InitialCondition=1  SampleTime=Ts  HasFrameUpgradeWarning=on
  V0 : Constant  Value=0
  Vdc_ref (V) : Constant  Value=Vdc_nom
  dq0 to abc : powerlib_meascontrol/Transformations/dq0 to abc  Alignment=90 degrees behind phase A axis
  Uctrl_inverter : Outport
  wires:
  Theta_PLL/1 -> dq0 to abc/2
  INT/1(Out) -> [iq_ref], Sum4/2
  Qref/1 -> Sum2/1
  Vdc_ref (V)/1 -> Sum7/1
  Sum8/1 -> Sum9/2
  Sum5/1 -> Sum3/1
  0-Mod_index_max/1 -> Polar to Cartesian/1
  Idq_gc/1 -> Demux/1
  dq0 to abc/1 -> Uctrl_inverter/1  "Uctrl"
  Mux/1 -> dq0 to abc/1  "Vdq0"
  Cartesian to Polar/2 -> Polar to Cartesian/2  "Phase"
  V0/1 -> Mux/3
  Polar to Cartesian/1 -> Mux/1
  Polar to Cartesian/2 -> Mux/2
  Sum9/1 -> Cartesian to Polar/2  "Vq inverter"
  Sum3/1 -> Cartesian to Polar/1  "Vd inverter"
  [Vdc] -> Avoid division by zero/1
  Cartesian to Polar/1 -> Product4/1
  Avoid division by zero/1 -> Product4/3
  K/1 -> Product4/2
  Product4/1 -> 0-Mod_index_max/1  "m"
  [Vd] -> Sum5/1
  [Vq] -> Sum8/3
  Demux4/2 -> [Vq]
  Demux4/1 -> [Vd]
  w_pu/1 -> [w_pu]
  Demux3/2 -> Sum9/1  "vq'"
  Demux3/1 -> Sum3/2  "vd'"
  [id_ref] -> Product1/1
  [iq_ref] -> Product3/1
  [id_ref] -> Product2/2
  [iq_ref] -> Product/3
  [w_pu] -> Product/2
  [w_pu] -> Product1/3
  Sum4/1 -> Mux2/2
  Sum6/1 -> Mux2/1
  Product3/1 -> Sum8/1
  Product2/1 -> Sum5/3
  Product1/1 -> Sum8/2
  Constant6/1 -> Product3/2
  Constant5/1 -> Product2/1
  Product/1 -> Sum5/2
  Demux/1 -> Sum6/2  "Id"
  Demux/2 -> Sum4/1  "Iq"
  Constant1/1 -> Product/1
  Mux2/1 -> Discrete PI Controller1/1(Error)
  Discrete PI Controller1/1(Out) -> Demux3/1
  Constant4/1 -> Product1/2
  First-Order Filter/1 -> INT/1(Max), Gain/1
  Math Function/1 -> Sum1/1
  Imax^2/1 -> Sum1/2
  Sum1/1 -> Math Function1/1
  Math Function1/1 -> First-Order Filter/1
  Unit Delay1/1 -> Discrete-Time Integrator1/2
  Sum2/1 -> Discrete-Time Integrator1/1
  Qmeas/1 -> Sum2/2
  Vmeas/1 -> Sum/2, Unit Delay1/1
  Discrete-Time Integrator1/1 -> Sum/1  "Vref"
  Constant3/1 -> INT/4(Ki)
  Gain/1 -> INT/2(Min)
  Data Type Conversion2/1 -> INT/6(Reset), INT/5(Hold)
  Constant2/1 -> INT/7(Reset Value), Data Type Conversion2/1
  Sum/1 -> INT/3(In)
  Discrete PI Controller/1(Out) -> Sum6/1, [id_ref], Math Function/1
  ->pu/1 -> Discrete PI Controller/1(Error)
  Sum7/1 -> ->pu/1
  Vdq_grid/1 -> Demux4/1
  Vdc/1 -> Sum7/2, [Vdc]

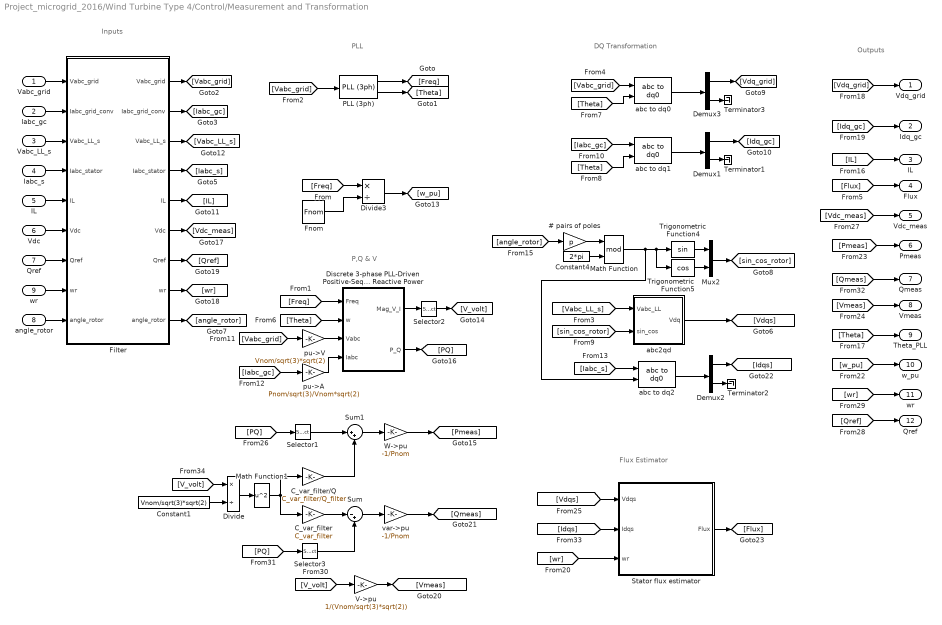
== system Project_microgrid_2016/Wind Turbine Type 4/Control/Measurement and Transformation ==
  note: Inputs
  note: P,Q & V
  note: DQ Transformation
  note: PLL
  note: Outputs
  note: Flux Estimator
  Vabc_grid : Inport
  Iabc_gc : Inport  Port=2
  Vabc_LL_s : Inport  Port=3
  Iabc_s : Inport  Port=4
  IL : Inport  Port=5
  Vdc : Inport  Port=6
  Qref : Inport  Port=7
  angle_rotor : Inport  Port=8
  wr : Inport  Port=9
  # pairs of poles : Gain  Gain=p  SaturateOnIntegerOverflow=on  OutDataTypeStr=Inherit: Same as input  ParamDataTypeStr=Inherit: Same as input
  C_var_filter : Gain  Gain=C_var_filter  SaturateOnIntegerOverflow=on  OutDataTypeStr=Inherit: Same as input  ParamDataTypeStr=Inherit: Same as input
  C_var_filter/Q : Gain  Gain=C_var_filter/Q_filter  SaturateOnIntegerOverflow=on  OutDataTypeStr=Inherit: Same as input  ParamDataTypeStr=Inherit: Same as input
  Constant1 : Constant  Value=Vnom/sqrt(3)*sqrt(2)
  Constant4 : Constant  Value=2*pi
  Demux1 : Demux  Outputs=[2 1]
  Demux2 : Demux  Outputs=[2 1]
  Demux3 : Demux  Outputs=[2 1]
  Discrete 3-phase PLL-Driven Positive-Sequence Active & Reactive Power : Subsystem  mask(Discrete 3-phase PLL-Driven Positive-Sequence Active & Reactive Power){Finit=Fnom, Fmin=Fnom*45/60, Par_Vinit=[Vnom/sqrt(3)*sqrt(2) 30], Par_Iinit=[Pnom/sqrt(3)/Vnom*sqrt(2) -10], Ts=Ts}
      mask prompts: Finit "Initial frequency (Hz):"; Fmin "Minimum frequency (Hz):"; Par_Vinit "Voltage initial input: [ Mag  Phase(Degrees) ]"; Par_Iinit "Current initial input: [ Mag  Phase(Degrees) ]"; Ts "Sample time:"
      mask help:
      | This discrete block measures the 3-phase active power P and reactive power Q  associated with a periodic set of 3-phase voltages and currents which may contain harmonics. P and Q are calculated by evaluating the fundamental values (positive-sequence) of the input voltages and currents with a running window over one cycle of the specified frequency (port Freq).
      |  Input port "Sin_Cos" (a two-dimension signal) provides the reference frame required for the computation.
      |
      | input 1: must give the frequency of the fundamental (Hz)
      | Input 2: must contain a  [sin(wt)  cos(wt)] two dimension signal , where w is the rotation speed (rad/s) of the reference frame used for the computation..
      | input 3: Vectorized 3-phase  instantaneous voltage (Vabc)
      | input 4: Vectorized 3-phase instantaneous current (Iabc)
      |
      | Output 1: Vector [Mag_V Mag_I] of the fundamental values (Magnitude) of the voltage & current (peak values of the positive-sequence)
      | Output 2: 3-phase PQ measurement vector [P(W) Q (var)] evaluated at the specified frequency. Current flowing into an RL circuit will produce  positive active and reactive powers.
      |
      | For the first cycle of simulation, the outputs are held constant using the values specified by the parameters "Initial input".
      | he value of the parameter "Minimum frequency" is used to determine the buffer size of the "Variable Transport Delay" block found inside this subsystem.
      mask init:
      | power_initmask();
      settings: OpenFcn=power_openblockproxy();
  Divide : Product  Inputs=*/
  Divide3 : Product  Inputs=*/
  Filter : Subsystem  mask{Freq=Freq_filter, Zeta=Zeta_filter, Ts=Ts}
      mask prompts: Freq "Cut-off frequency (Hz):"; Zeta "Damping factor Zeta:"; Ts "Sample time"
  Fnom : Constant  Value=Fnom
  Math Function : Math  Operator=mod  SaturateOnIntegerOverflow=on
  Math Function1 : Math  Operator=square  SaturateOnIntegerOverflow=on
  Mux2 : Mux  Inputs=2
  PLL (3ph) : powerlib_meascontrol/PLL/PLL (3ph)  Fmin=0.75*Fnom  Par_Init=[-45 Fnom]  ParK=[60 1400 1]  TcD=1e-4  MaxRateChangeFreq=12  FilterCutOffFreq=25  Ts=Ts  AGC=on
  Selector1 : Selector  InputPortWidth=2  IndexOptions=Index vector (dialog)  Indices=1  OutputSizes=1
  Selector2 : Selector  InputPortWidth=2  IndexOptions=Index vector (dialog)  Indices=1  OutputSizes=1
  Selector3 : Selector  InputPortWidth=2  IndexOptions=Index vector (dialog)  Indices=2  OutputSizes=1
  Stator flux estimator : Subsystem
  Sum : Sum  Inputs=|-+
  Sum1 : Sum  Inputs=|++
  Terminator1 : Terminator
  Terminator2 : Terminator
  Terminator3 : Terminator
  Trigonometric Function4 : Trigonometry
  Trigonometric Function5 : Trigonometry  Operator=cos
  V->pu : Gain  Gain=1/(Vnom/sqrt(3)*sqrt(2))  SaturateOnIntegerOverflow=on  OutDataTypeStr=Inherit: Same as input  ParamDataTypeStr=Inherit: Same as input
  W->pu : Gain  Gain=-1/Pnom  SaturateOnIntegerOverflow=on  OutDataTypeStr=Inherit: Same as input  ParamDataTypeStr=Inherit: Same as input
  abc to dq0 : powerlib_meascontrol/Transformations/abc to dq0  Alignment=90 degrees behind phase A axis
  abc to dq1 : powerlib_meascontrol/Transformations/abc to dq0  Alignment=90 degrees behind phase A axis
  abc to dq2 : powerlib_meascontrol/Transformations/abc to dq0  Alignment=90 degrees behind phase A axis
  abc2qd : Subsystem
  pu->A : Gain  Gain=Pnom/sqrt(3)/Vnom*sqrt(2)  SaturateOnIntegerOverflow=on  OutDataTypeStr=Inherit: Same as input  ParamDataTypeStr=Inherit: Same as input
  pu->V : Gain  Gain=Vnom/sqrt(3)*sqrt(2)  SaturateOnIntegerOverflow=on  OutDataTypeStr=Inherit: Same as input  ParamDataTypeStr=Inherit: Same as input
  "var->pu " : Gain  Gain=-1/Pnom  SaturateOnIntegerOverflow=on  OutDataTypeStr=Inherit: Same as input  ParamDataTypeStr=Inherit: Same as input
  Vdq_grid : Outport
  Idq_gc : Outport  Port=2
  "IL " : Outport  Port=3
  Flux : Outport  Port=4
  Vdc_meas : Outport  Port=5
  Pmeas : Outport  Port=6
  Qmeas : Outport  Port=7
  Vmeas : Outport  Port=8
  Theta_PLL : Outport  Port=9
  w_pu : Outport  Port=10
  "wr " : Outport  Port=11
  "Qref " : Outport  Port=12
  wires:
  Math Function/1 -> Trigonometric Function4/1, Trigonometric Function5/1, abc to dq2/2
  [IL] -> "IL "/1
  Filter/5("IL ") -> [IL]
  IL/1 -> Filter/5(IL)
  Sum1/1 -> W->pu/1
  C_var_filter/Q/1 -> Sum1/2
  Selector1/1 -> Sum1/1
  Math Function1/1 -> C_var_filter/1, C_var_filter/Q/1
  Sum/1 -> "var->pu "/1
  C_var_filter/1 -> Sum/1
  Selector3/1 -> Sum/2
  Divide/1 -> Math Function1/1
  Constant1/1 -> Divide/2
  [V_volt] -> Divide/1
  Filter/3("Vabc_LL_s ") -> [Vabc_LL_s]
  Vabc_LL_s/1 -> Filter/3(Vabc_LL_s)
  Iabc_s/1 -> Filter/4(Iabc_stator)
  Iabc_gc/1 -> Filter/2(Iabc_grid_conv)
  Filter/7("Qref ") -> [Qref]
  Filter/8("wr ") -> [wr]
  Filter/6("Vdc ") -> [Vdc_meas]
  Filter/4("Iabc_stator ") -> [Iabc_s]
  Filter/2("Iabc_grid_conv ") -> [Iabc_gc]
  Filter/1("Vabc_grid ") -> [Vabc_grid]
  wr/1 -> Filter/8(wr)
  Qref/1 -> Filter/7(Qref)
  Vdc/1 -> Filter/6(Vdc)
  Vabc_grid/1 -> Filter/1(Vabc_grid)
  Discrete 3-phase PLL-Driven Positive-Sequence Active & Reactive Power/2(P_Q) -> [PQ]
  [Iabc_gc] -> pu->A/1
  [Vabc_grid] -> pu->V/1
  [Flux] -> Flux/1
  [wr] -> "wr "/1
  [Qref] -> "Qref "/1
  [Vdc_meas] -> Vdc_meas/1
  [PQ] -> Selector1/1
  pu->A/1 -> Discrete 3-phase PLL-Driven Positive-Sequence Active & Reactive Power/4(Iabc)
  [Vmeas] -> Vmeas/1
  [Pmeas] -> Pmeas/1
  [w_pu] -> w_pu/1
  [Idq_gc] -> Idq_gc/1
  [Vdq_grid] -> Vdq_grid/1
  Demux1/1 -> [Idq_gc]
  [Theta] -> Theta_PLL/1
  [Iabc_gc] -> abc to dq1/1
  [Vabc_grid] -> PLL (3ph)/1
  [Theta] -> abc to dq1/2
  [Theta] -> abc to dq0/2
  [Theta] -> Discrete 3-phase PLL-Driven Positive-Sequence Active & Reactive Power/2(w)
  [Vabc_grid] -> abc to dq0/1
  PLL (3ph)/2 -> [Theta]
  [Freq] -> Discrete 3-phase PLL-Driven Positive-Sequence Active & Reactive Power/1(Freq)
  [Freq] -> Divide3/1
  W->pu/1 -> [Pmeas]
  pu->V/1 -> Discrete 3-phase PLL-Driven Positive-Sequence Active & Reactive Power/3(Vabc)
  Divide3/1 -> [w_pu]
  Fnom/1 -> Divide3/2
  PLL (3ph)/1 -> [Freq]
  abc to dq0/1 -> Demux3/1
  abc to dq1/1 -> Demux1/1
  Demux3/2 -> Terminator3/1
  Demux3/1 -> [Vdq_grid]
  Demux1/2 -> Terminator1/1
  Discrete 3-phase PLL-Driven Positive-Sequence Active & Reactive Power/1(Mag_V_I) -> Selector2/1
  Selector2/1 -> [V_volt]
  [V_volt] -> V->pu/1
  V->pu/1 -> [Vmeas]
  [PQ] -> Selector3/1
  "var->pu "/1 -> [Qmeas]
  [Qmeas] -> Qmeas/1
  [wr] -> Stator flux estimator/3(wr)
  [Idqs] -> Stator flux estimator/2(Idqs)
  [Vdqs] -> Stator flux estimator/1(Vdqs)
  [Iabc_s] -> abc to dq2/1
  abc to dq2/1 -> Demux2/1
  Demux2/2 -> Terminator2/1
  Demux2/1 -> [Idqs]
  Mux2/1 -> [sin_cos_rotor]
  [sin_cos_rotor] -> abc2qd/2(sin_cos)
  [Vabc_LL_s] -> abc2qd/1(Vabc_LL)
  [angle_rotor] -> # pairs of poles/1
  Trigonometric Function4/1 -> Mux2/1
  Trigonometric Function5/1 -> Mux2/2
  abc2qd/1(Vdq) -> [Vdqs]
  Constant4/1 -> Math Function/2
  # pairs of poles/1 -> Math Function/1
  Stator flux estimator/1(Flux) -> [Flux]
  angle_rotor/1 -> Filter/9(angle_rotor)
  Filter/9("angle_rotor ") -> [angle_rotor]

== system Project_microgrid_2016/Wind Turbine Type 4/Control/Pulse Generator ==
  Duty_Cycle : Inport
  Add : Sum  Inputs=-+
  Constant3 : Constant
  Constant4 : Constant  Value=0
  Digital Clock : DigitalClock  SampleTime=Ts
  Divide2 : Product  Inputs=**
  Divide3 : Product  Inputs=**
  Math Function : Math  Operator=mod  SaturateOnIntegerOverflow=on
  Nb_of_samples_by_cycle : Constant  Value=1/Freq_sawtooth/Ts
  Relational Operator1 : RelationalOperator  Operator=>  OutDataTypeStr=boolean
  Rounding Function1 : Rounding  Operator=round
  Switch : Switch  Threshold=0.5
  Ts : Constant  Value=Ts
  Pulse : Outport
  wires:
  Math Function/1 -> Relational Operator1/2
  Constant4/1 -> Switch/3
  Constant3/1 -> Switch/1
  Relational Operator1/1 -> Switch/2
  Nb_of_samples_by_cycle/1 -> Rounding Function1/1
  Divide2/1 -> Relational Operator1/1
  Divide3/1 -> Add/2, Math Function/2  "Period_of_cycle"
  Duty_Cycle/1 -> Divide2/1
  Rounding Function1/1 -> Divide3/2  "Nb_of_samples_by_cycle"
  Ts/1 -> Divide3/1, Add/1
  Digital Clock/1 -> Math Function/1
  Add/1 -> Divide2/2
  Switch/1 -> Pulse/1
